simulink model "q2_part_d_continous"  (R2020b)
settings: Solver=VariableStepAuto  StartTime=0.0  StopTime=1.8e5  RelTol=0.5e-3
model workspace (MATLAB code in the model file):
  | G11 = tf(tfs.NUM(1,1),tfs.DEN(1,1),Ts);
  | G12 = tf(tfs.NUM(2,1),tfs.DEN(2,1),Ts);
  | G13 = tf(tfs.NUM(3,1),tfs.DEN(3,1),Ts);
  | G21 = tf(tfs.NUM(1,2),tfs.DEN(1,2),Ts);
  | G22 = tf(tfs.NUM(2,2),tfs.DEN(2,2),Ts);
  | G23 = tf(tfs.NUM(3,2),tfs.DEN(3,2),Ts);
values from neighbouring files (symbols this model uses):
  tfs = tf(sys)    [q2_a_and_b.m]
  Ts = tout(2) - tout(1)    [q2_a_and_b.m]
libraries: cstblocks x1, pid_lib x1
settings Model: OrderedModelArguments=off  Creator=Jamesh  LastModifiedBy=HP
settings SolverCC: AlgebraicLoopSolver=LineSearch

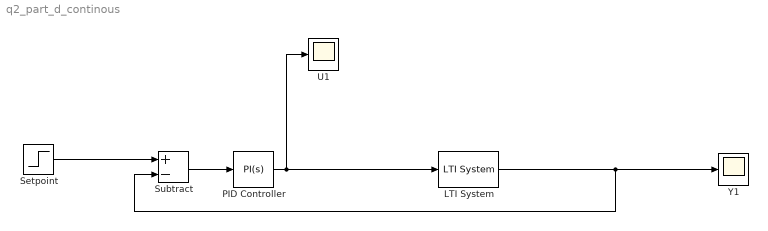
== system q2_part_d_continous ==
  LTI System : cstblocks/LTI System  sys=G11  IC=[]
  PID Controller : pid_lib/PID Controller  Controller=PI  Form=Parallel  TimeDomain=Continuous-time  UseExternalTs=off  SampleTime=Ts  IntegratorMethod=Forward Euler  FilterMethod=Forward Euler  ControllerParametersSource=internal  P=179.074373920372  I=5.21380137768688e-05  D=0  UseFilter=on  N=9.78953011712136e-05  TunerSelectOption=Transfer Function Based (PID Tuner App)  InitialConditionSource=internal  InitialConditionForIntegrator=0  InitialConditionForFilter=0  DifferentiatorICPrevScaledInput=0  ExternalReset=none  TrackingMode=off  Kt=1  LimitOutput=off  SatLimitsSource=internal  UpperSaturationLimit=inf  LowerSaturationLimit=-inf  LinearizeAsGain=on  AntiWindupMode=none  Kb=1  POutMin=[]  POutMax=[]  IOutMin=[]  IOutMax=[]  DOutMin=[]  DOutMax=[]  NOutMin=[]  NOutMax=[]  SumOutMin=[]  SumOutMax=[]  SaturationOutMin=[]  SaturationOutMax=[]  PParamMin=[]  PParamMax=[]  IParamMin=[]  IParamMax=[]  DParamMin=[]  DParamMax=[]  NParamMin=[]  NParamMax=[]  KbParamMin=[]  KbParamMax=[]  KtParamMin=[]  KtParamMax=[]  KbOutMin=[]  KbOutMax=[]  KtOutMin=[]  KtOutMax=[]  IntegratorOutMin=[]  IntegratorOutMax=[]  FilterOutMin=[]  FilterOutMax=[]  SumI1OutMin=[]  SumI1OutMax=[]  SumI2OutMin=[]  SumI2OutMax=[]  SumI3OutMin=[]  SumI3OutMax=[]  SumI4OutMin=[]  SumI4OutMax=[]  SumDOutMin=[]  SumDOutMax=[]  DifferentiatorOutMin=[]  DifferentiatorOutMax=[]  FilterDiffOutCoefMin=[]  FilterDiffOutCoefMax=[]  ReciprocalOutMin=[]  ReciprocalOutMax=[]  SumDenOutMin=[]  SumDenOutMax=[]  SumNumOutMin=[]  SumNumOutMax=[]  DivideOutMin=[]  DivideOutMax=[]  UdiffTsProdOutMin=[]  UdiffTsProdOutMax=[]  NTsProdOutMin=[]  NTsProdOutMax=[]  UintegralTsProdOutMin=[]  UintegralTsProdOutMax=[]  UngainTsProdOutMin=[]  UngainTsProdOutMax=[]  IntegratorContinuousStateAttributes=''  IntegratorStateMustResolveToSignalObject=off  IntegratorRTWStateStorageClass=Auto  FilterContinuousStateAttributes=''  FilterStateMustResolveToSignalObject=off  FilterRTWStateStorageClass=Auto  ParallelPVariant=InternalParameters  IdealPVariant=Disabled  IVariant=InternalParameters  DVariant=Disabled  IntegratorVariant=Continuous  SatVariant=Disabled  AWVariant=Passthrough  PCopyVariant=Disabled  TRVariant=Disabled  FdbkBlocksVariant=Forward  IdealPFdbkVariant=Disabled  SatFdbkVariant=Disabled  DerivativeFilterVariant=Disabled  NVariant=Disabled  NCopyVariant=Disabled_SignalSpec  FilterICVariant=Disabled  IntegratorICVariant=InternalICs  ExternalResetVariant=Disabled  TRSumVariant=Passthrough  SumFdbkVariant=Disabled  SumVariant=Sum_PI  TsampFilterVariant=InternalTs  TsampNgainVariant=Passthrough  TsampIntegralVariant=Passthrough  ExternalSaturationOutDataTypeStr=Inherit: Same as second input
  Setpoint : Step  SampleTime=0
  Subtract : Sum  Inputs=+-
  U1 : Scope
  Y1 : Scope
  wires:
  PID Controller/1 -> LTI System/1, U1/1
  Setpoint/1 -> Subtract/1
  Subtract/1 -> PID Controller/1
  LTI System/1 -> Subtract/2, Y1/1
